simulink model "RPfrhyb1"  (R2020a)
settings: Solver=ode45  StartTime=0.0  StopTime=8  MaxStep=1e-3  RelTol=1e-6  AbsTol=1e-6
InitFcn:
  | k = 0.9;
  | m = 1.5;
  | l = 1;
  | g = 9.81;
  | phi0 = pi/4;
  | phi_dot0 = 15;
libraries: simulink x1
settings Model: Creator=Home  LastModifiedBy=peter

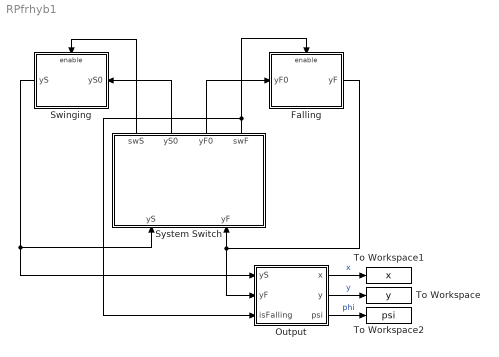
== system RPfrhyb1 ==
  Falling : Subsystem
  Output : Subsystem  mask{psiEnd=pi/10}
      mask prompts: psiEnd "maximal amplitude for termination:"
  Swinging : Subsystem
  System Switch : Subsystem
  To Workspace : ToWorkspace  VariableName=y  SaveFormat=Timeseries  SampleTime=-1
  To Workspace1 : ToWorkspace  VariableName=x  SaveFormat=Timeseries  SampleTime=-1
  To Workspace2 : ToWorkspace  VariableName=psi  SaveFormat=Timeseries  SampleTime=-1
  wires:
  Swinging/1(yS) -> Output/1(yS), System Switch/1(yS)
  Falling/1(yF) -> Output/2(yF), System Switch/2(yF)
  Output/3(psi) -> To Workspace2/1  "phi"
  Output/2(y) -> To Workspace/1  "y"
  Output/1(x) -> To Workspace1/1  "x"
  System Switch/4(swF) -> Falling/Enable, Output/3(isFalling)
  System Switch/1(swS) -> Swinging/Enable
  System Switch/2(yS0) -> Swinging/1(yS0)
  System Switch/3(yF0) -> Falling/1(yF0)

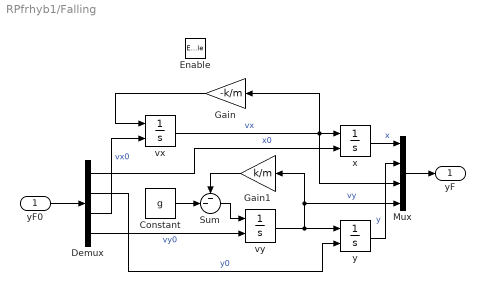
== system RPfrhyb1/Falling ==
  yF0 : Inport
  Enable : EnablePort  StatesWhenEnabling=reset
  Constant : Constant  Value=g
  Demux : Demux
  Gain : Gain  Gain=-k/m
  Gain1 : Gain  Gain=k/m
  Mux : Mux
  Sum : Sum  Inputs=--|
  vx : Integrator  InitialConditionSource=external
  vy : Integrator  InitialConditionSource=external
  x : Integrator  InitialConditionSource=external
  y : Integrator  InitialConditionSource=external
  yF : Outport
  wires:
  vx/1 -> x/1, Gain/1, Mux/3  "vx"
  Gain/1 -> vx/1
  x/1 -> Mux/1  "x"
  Gain1/1 -> Sum/1
  Demux/4 -> vy/2  "vy0"
  vy/1 -> Mux/4, Gain1/1, y/1  "vy"
  Sum/1 -> vy/1
  Constant/1 -> Sum/2
  Demux/2 -> y/2  "y0"
  Demux/1 -> x/2  "x0"
  Demux/3 -> vx/2  "vx0"
  yF0/1 -> Demux/1
  y/1 -> Mux/2  "y"
  Mux/1 -> yF/1

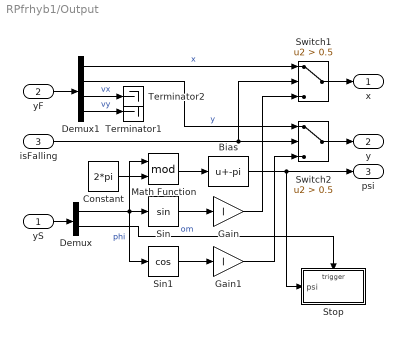
== system RPfrhyb1/Output ==
  yS : Inport
  yF : Inport  Port=2
  isFalling : Inport  Port=3
  Bias : Bias  Bias=-pi
  Constant : Constant  Value=2*pi
  Demux : Demux  Outputs=2
  Demux1 : Demux
  Gain : Gain  Gain=l
  Gain1 : Gain  Gain=l
  Math Function : Math  Operator=mod  SaturateOnIntegerOverflow=on
  Sin : Trigonometry
  Sin1 : Trigonometry  Operator=cos
  Stop : Subsystem  TreatAsAtomicUnit=on
  Switch1 : Switch  Criteria=u2 > Threshold  Threshold=0.5
  Switch2 : Switch  Criteria=u2 > Threshold  Threshold=0.5
  Terminator1 : Terminator
  Terminator2 : Terminator
  x : Outport
  y : Outport  Port=2
  psi : Outport  Port=3
  wires:
  yS/1 -> Demux/1
  yF/1 -> Demux1/1
  Switch1/1 -> x/1
  Switch2/1 -> y/1
  isFalling/1 -> Switch2/2, Switch1/2
  Demux1/1 -> Switch1/1  "x"
  Demux1/2 -> Switch2/1  "y"
  Demux/1 -> Sin1/1, Math Function/1, Sin/1  "phi"
  Sin/1 -> Gain/1
  Gain/1 -> Switch1/3
  Sin1/1 -> Gain1/1
  Gain1/1 -> Switch2/3
  Constant/1 -> Math Function/2
  Math Function/1 -> Bias/1
  Bias/1 -> psi/1, Stop/1(psi)
  Demux/2 -> Stop/Trigger  "om"
  Demux1/4 -> Terminator1/1  "vy"
  Demux1/3 -> Terminator2/1  "vx"

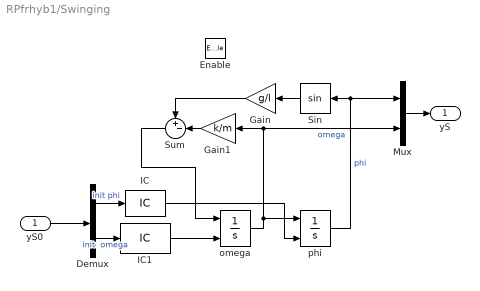
== system RPfrhyb1/Swinging ==
  yS0 : Inport
  Enable : EnablePort  StatesWhenEnabling=reset
  Demux : Demux  Outputs=2
  Gain : Gain  Gain=g/l
  Gain1 : Gain  Gain=k/m
  IC : InitialCondition  Value=phi0
  IC1 : InitialCondition  Value=phi_dot0
  Mux : Mux  Inputs=2
  Sin : Trigonometry
  Sum : Sum  Inputs=+-|
  omega : Integrator  InitialConditionSource=external  InitialCondition=phi_dot0
  phi : Integrator  InitialConditionSource=external  InitialCondition=phi0
  yS : Outport
  wires:
  phi/1 -> Sin/1, Mux/1  "phi"
  Sum/1 -> omega/1
  omega/1 -> Gain1/1, Mux/2, phi/1  "omega"
  Gain/1 -> Sum/1
  Sin/1 -> Gain/1
  IC/1 -> phi/2
  IC1/1 -> omega/2
  Mux/1 -> yS/1
  yS0/1 -> Demux/1
  Demux/2 -> IC1/1  "init  omega"
  Demux/1 -> IC/1  "init phi"
  Gain1/1 -> Sum/2

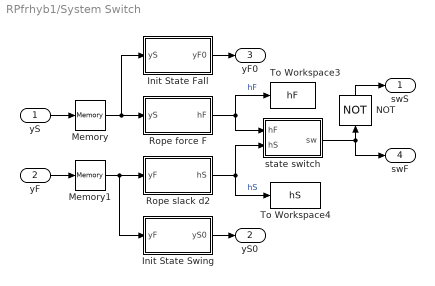
== system RPfrhyb1/System Switch ==
  yS : Inport
  yF : Inport  Port=2
  Init State Fall : Subsystem
  Init State Swing : Subsystem
  Memory : Memory
  Memory1 : Memory
  NOT : Logic  Operator=NOT  IconShape=distinctive  AllPortsSameDT=off  OutDataTypeStr=boolean
  Rope force F : Subsystem
  Rope slack d2 : Subsystem
  To Workspace3 : ToWorkspace  VariableName=hF  SaveFormat=Timeseries  SampleTime=-1
  To Workspace4 : ToWorkspace  VariableName=hS  SaveFormat=Timeseries  SampleTime=-1
  state switch : Subsystem
  swS : Outport
  yS0 : Outport  Port=2
  yF0 : Outport  Port=3
  swF : Outport  Port=4
  wires:
  Rope slack d2/1(hS) -> To Workspace4/1, state switch/2(hS)  "hS"
  NOT/1 -> swS/1
  Memory1/1 -> Rope slack d2/1(yF), Init State Swing/1(yF)
  Rope force F/1(hF) -> To Workspace3/1, state switch/1(hF)  "hF"
  yS/1 -> Memory/1
  Memory/1 -> Rope force F/1(yS), Init State Fall/1(yS)
  yF/1 -> Memory1/1
  Init State Fall/1(yF0) -> yF0/1
  state switch/1(sw) -> swF/1, NOT/1
  Init State Swing/1(yS0) -> yS0/1

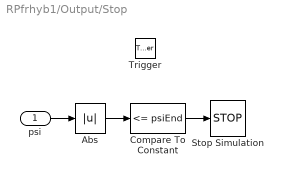
== system RPfrhyb1/Output/Stop ==
  psi : Inport
  Trigger : TriggerPort  TriggerType=either  VariantControl=Variant
  Abs : Abs
  Compare To Constant : simulink/Logic and Bit Operations/Compare To Constant  relop=<=  const=psiEnd  OutDataTypeStr=boolean
  Stop Simulation : Stop
  wires:
  psi/1 -> Abs/1
  Compare To Constant/1 -> Stop Simulation/1
  Abs/1 -> Compare To Constant/1

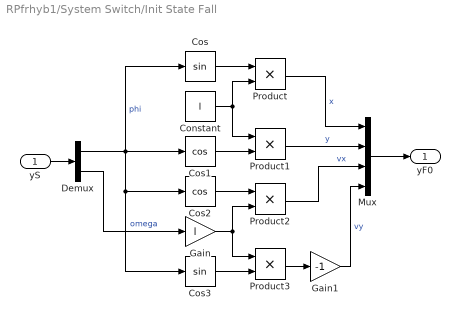
== system RPfrhyb1/System Switch/Init State Fall ==
  yS : Inport
  Constant : Constant  Value=l
  Cos : Trigonometry
  Cos1 : Trigonometry  Operator=cos
  Cos2 : Trigonometry  Operator=cos
  Cos3 : Trigonometry
  Demux : Demux  Outputs=2
  Gain : Gain  Gain=l
  Gain1 : Gain  Gain=-1
  Mux : Mux
  Product{,1..3} (4 alike) : Product
  yF0 : Outport
  wires:
  Product/1 -> Mux/1  "x"
  Cos/1 -> Product/1
  Constant/1 -> Product/2, Product1/1
  Product1/1 -> Mux/2  "y"
  Cos1/1 -> Product1/2
  Demux/1 -> Cos/1, Cos2/1, Cos3/1, Cos1/1  "phi"
  yS/1 -> Demux/1
  Mux/1 -> yF0/1
  Cos3/1 -> Product3/2
  Demux/2 -> Gain/1  "omega"
  Cos2/1 -> Product2/1
  Gain/1 -> Product2/2, Product3/1
  Product2/1 -> Mux/3  "vx"
  Product3/1 -> Gain1/1
  Gain1/1 -> Mux/4  "vy"

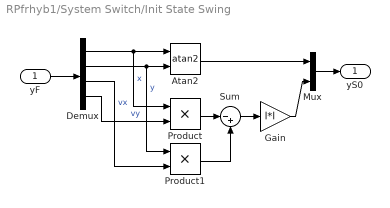
== system RPfrhyb1/System Switch/Init State Swing ==
  yF : Inport
  Atan2 : Trigonometry  Operator=atan2
  Demux : Demux
  Gain : Gain  Gain=l*l
  Mux : Mux  Inputs=2
  Product : Product
  Product1 : Product
  Sum : Sum  Inputs=|-+
  yS0 : Outport
  wires:
  yF/1 -> Demux/1
  Mux/1 -> yS0/1
  Demux/1 -> Product/1, Atan2/1  "x"
  Demux/2 -> Product1/1, Atan2/2  "y"
  Atan2/1 -> Mux/1
  Demux/4 -> Product/2  "vy"
  Demux/3 -> Product1/2  "vx"
  Product1/1 -> Sum/2
  Product/1 -> Sum/1
  Sum/1 -> Gain/1
  Gain/1 -> Mux/2

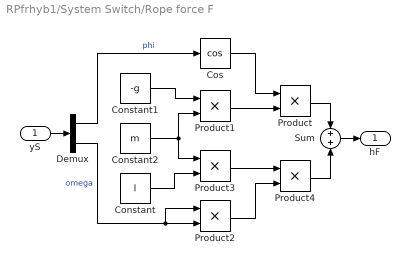
== system RPfrhyb1/System Switch/Rope force F ==
  yS : Inport
  Constant : Constant  Value=l
  Constant1 : Constant  Value=-g
  Constant2 : Constant  Value=m
  Cos : Trigonometry  Operator=cos
  Demux : Demux  Outputs=2
  Product{,1..4} (5 alike) : Product
  Sum : Sum
  hF : Outport
  wires:
  Constant1/1 -> Product1/1
  Constant2/1 -> Product3/1, Product1/2
  Product/1 -> Sum/1
  Demux/2 -> Product2/1, Product2/2  "omega"
  Product1/1 -> Product/2
  Cos/1 -> Product/1
  Constant/1 -> Product3/2
  Product3/1 -> Product4/1
  Product2/1 -> Product4/2
  Product4/1 -> Sum/2
  Sum/1 -> hF/1
  yS/1 -> Demux/1
  Demux/1 -> Cos/1  "phi"

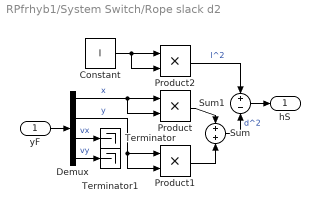
== system RPfrhyb1/System Switch/Rope slack d2 ==
  yF : Inport
  Constant : Constant  Value=l
  Demux : Demux
  Product : Product
  Product1 : Product
  Product2 : Product
  Sum : Sum
  Sum1 : Sum  Inputs=+-
  Terminator : Terminator
  Terminator1 : Terminator
  hS : Outport
  wires:
  Demux/4 -> Terminator1/1  "vy"
  Product2/1 -> Sum1/1  "l^2"
  Demux/2 -> Product1/2, Product1/1  "y"
  Demux/1 -> Product/2, Product/1  "x"
  Product/1 -> Sum/1
  Demux/3 -> Terminator/1  "vx"
  Sum/1 -> Sum1/2  "d^2"
  yF/1 -> Demux/1
  Sum1/1 -> hS/1
  Product1/1 -> Sum/2
  Constant/1 -> Product2/2, Product2/1

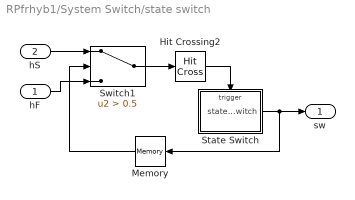
== system RPfrhyb1/System Switch/state switch ==
  hF : Inport
  hS : Inport  Port=2
  Hit Crossing2 : HitCross  HitCrossingDirection=falling
  Memory : Memory
  State Switch : Subsystem
  Switch1 : Switch  Criteria=u2 > Threshold  Threshold=0.5
  sw : Outport
  wires:
  Hit Crossing2/1 -> State Switch/Trigger
  State Switch/1(state switch) -> sw/1, Memory/1
  Switch1/1 -> Hit Crossing2/1
  Memory/1 -> Switch1/2
  hS/1 -> Switch1/1
  hF/1 -> Switch1/3

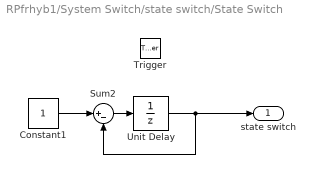
== system RPfrhyb1/System Switch/state switch/State Switch ==
  Trigger : TriggerPort  TriggerType=falling  VariantControl=Variant  InitialTriggerSignalState=positive  PortDimensions=1
  Constant1 : Constant
  Sum2 : Sum  Inputs=|+-
  Unit Delay : UnitDelay  SampleTime=-1  HasFrameUpgradeWarning=on
  state switch : Outport  VectorParamsAs1DForOutWhenUnconnected=off
  wires:
  Constant1/1 -> Sum2/1
  Sum2/1 -> Unit Delay/1
  Unit Delay/1 -> state switch/1, Sum2/2
